simulink model "primary_node"  (Simulink 7.8)
settings: Solver=FixedStepDiscrete  SolverMode=SingleTasking  StartTime=0.0  StopTime=10.0  FixedStep=0.01  RelTol=1e-3
InitFcn:
  | clear all
  | missions
  | common
  | physical_constants
  | initial_values
  | l2plus
values from neighbouring files (symbols this model uses):
  InitialPoint = 0    [l2plus.m]
  IPStar = 0    [l2plus.m]
  lla_ltp_gain = [r * (pi / 180 / 1e7); v * cos(ref_lla(1)) * (pi / 180 / 1e7); 1e-6]    [common.m]
  MaxDwnPthStar = 1    [l2plus.m]
  ref_lla_sense = int32([36.963765 * 1e7; -122.00191 * 1e7; 0 * 1e6])    [common.m]
  switchDistance = 4    [l2plus.m]
  T_step = 0.01    [common.m]
  tanIntercept = tan( 45*pi/180 )    [l2plus.m]
  TStar = single(2)    [l2plus.m]
  Turn2Track = 0    [l2plus.m]
  wheelbase = 3.27    [physical_constants.m]
undefined symbols (not defined in the file or in its folder): ANmax, ClearGpsData, ClearRudderAngle, cpInitCommunications, DiscIntNeverNeededParam, GetGpsDataPacked, GetRcNodeAvailability, GetThrottleDataPacked, Init_onlyOnce, Init_Reset, MatlabGetMavLinkManualControl, MavLinkEvaluateMissionState, MavLinkEvaluateParameterState, MavLinkReceive, MavLinkScheduleCurrentMission, MavLinkScheduleGpsOrigin, MavLinkTransmit, NodeTransmitStatus, PrimaryNodeInit, RudderSendAngleCommand, SendThrottleCommand, test_waypoints, u1, u2, y1
libraries: dsPICdrivers x32, uSimLib x21, simulink x19, ecan_dspic x2, etargetslib x2, simulink_need_slupdate x1
(part 2 of 2)

== system primary_node/Sensor Inputs/Update CPU Load ==
  Calculus Time Step : dsPICdrivers/OTHERS/Calculus Time Step  Tag=dsPIC_CalculusTimeStep  SampleTime=1  PR1chk=on
  Compare To Zero : simulink/Logic and Bit Operations/Compare To Zero  relop=~=  OutDataTypeStr=uint8
  Constant : Constant
  Data Store Write : DataStoreWrite  DataStoreName=nodeCpuLoad
  Data Type Conversion6 : DataTypeConversion  OutDataTypeStr=single
  Data Type Conversion7 : DataTypeConversion  OutDataTypeStr=single
  Gain : Gain  Gain=100  OutDataTypeStr=uint8
  Product : Product  Inputs=*/  RndMeth=Zero
  Switch : Switch  Criteria=u2 ~= 0
  wires:
  Calculus Time Step/1 -> Data Type Conversion6/1
  Calculus Time Step/2 -> Data Type Conversion7/1
  Product/1 -> Gain/1
  Gain/1 -> Data Store Write/1
  Data Type Conversion6/1 -> Product/1
  Data Type Conversion7/1 -> Switch/1, Compare To Zero/1
  Switch/1 -> Product/2
  Compare To Zero/1 -> Switch/2
  Constant/1 -> Switch/3

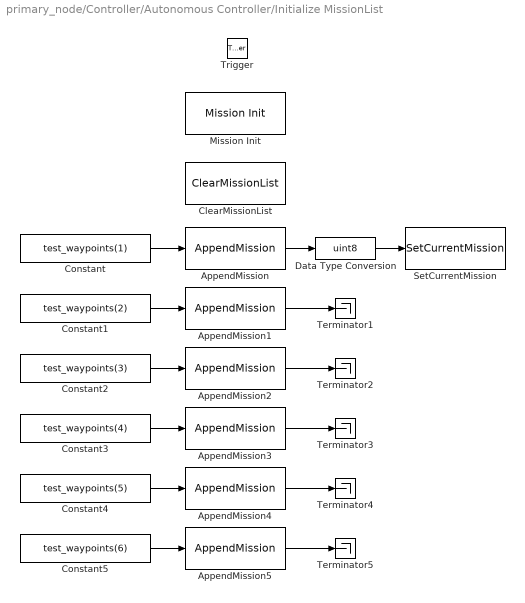
== system primary_node/Controller/Autonomous Controller/Initialize MissionList ==
  Trigger : TriggerPort  TriggerType=falling  PortDimensions=1
  AppendMission{,1..5} (6 alike) : uSimLib/Mission Manager/AppendMission  sampleTime=-1
  ClearMissionList : uSimLib/Mission Manager/ClearMissionList  Priority=1  sampleTime=-1
      link override Data Store Write1: DataStoreElements=mList.updated
  Constant : Constant  Value=test_waypoints(1)  OutDataTypeStr=Bus: Mission
  Constant1 : Constant  Value=test_waypoints(2)  OutDataTypeStr=Bus: Mission
  Constant2 : Constant  Value=test_waypoints(3)  OutDataTypeStr=Bus: Mission
  Constant3 : Constant  Value=test_waypoints(4)  OutDataTypeStr=Bus: Mission
  Constant4 : Constant  Value=test_waypoints(5)  OutDataTypeStr=Bus: Mission
  Constant5 : Constant  Value=test_waypoints(6)  OutDataTypeStr=Bus: Mission
  Data Type Conversion : DataTypeConversion  OutDataTypeStr=uint8
  Mission Init : uSimLib/Mission Manager/Mission Init  Priority=0  maxMissions=16  sampleTime=-1
      link override Data Store Write: SampleTime=-1
  SetCurrentMission : uSimLib/Mission Manager/SetCurrentMission  sampleTime=-1
  Terminator{1..5} (5 alike) : Terminator
  wires:
  Data Type Conversion/1 -> SetCurrentMission/1
  Constant5/1 -> AppendMission5/1
  AppendMission5/1 -> Terminator5/1
  Constant4/1 -> AppendMission4/1
  AppendMission4/1 -> Terminator4/1
  Constant3/1 -> AppendMission3/1
  AppendMission3/1 -> Terminator3/1
  Constant2/1 -> AppendMission2/1
  AppendMission2/1 -> Terminator2/1
  Constant1/1 -> AppendMission1/1
  AppendMission1/1 -> Terminator1/1
  Constant/1 -> AppendMission/1
  AppendMission/1 -> Data Type Conversion/1

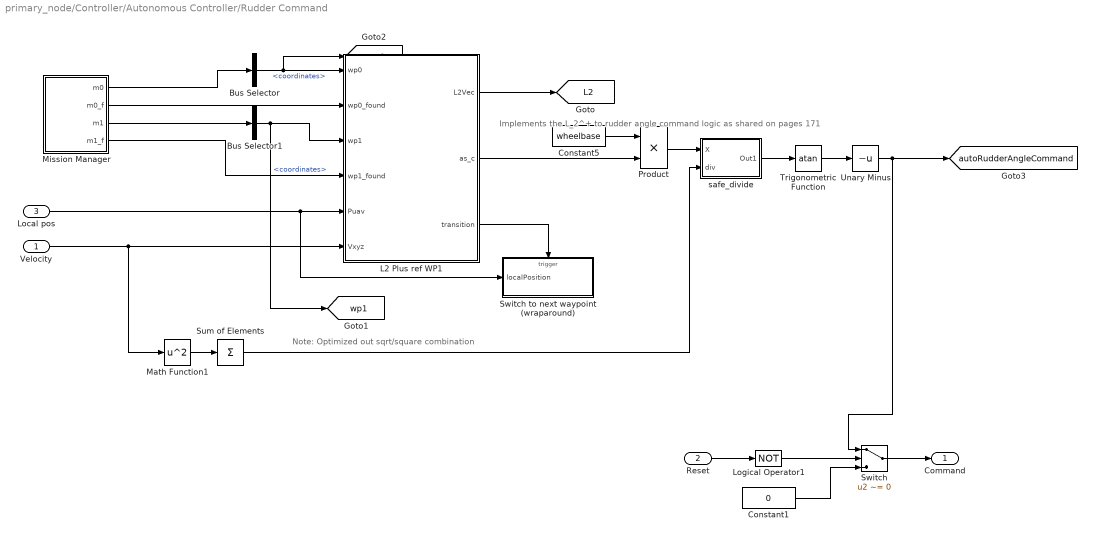
== system primary_node/Controller/Autonomous Controller/Rudder Command ==
  note: Implements the L_2^+ to rudder angle command logic as shared on pages 171
  note: Note: Optimized out sqrt/square combination
  Velocity : Inport
  Reset : Inport  Port=2
  Local pos : Inport  Port=3
  Bus Selector : BusSelector  OutputSignals=coordinates
  Bus Selector1 : BusSelector  OutputSignals=coordinates
  Constant1 : Constant  Value=0  OutDataTypeStr=single
  Constant5 : Constant  Value=wheelbase  OutDataTypeStr=boolean
  L2 Plus ref WP1 : MATLAB Function  TreatAsAtomicUnit=on
  Logical Operator1 : Logic  Operator=NOT  Inputs=1  AllPortsSameDT=off  OutDataTypeStr=boolean
  Math Function1 : Math  Operator=square  SaturateOnIntegerOverflow=on
  Mission Manager : Subsystem
  Product : Product  Inputs=**  RndMeth=Zero
  Sum of Elements : Sum  Inputs=+
  Switch : Switch  Criteria=u2 ~= 0
  Switch to next waypoint (wraparound) : Subsystem  TreatAsAtomicUnit=on
  Trigonometric Function : Trigonometry  Operator=atan
  Unary Minus : UnaryMinus
  safe_divide : Subsystem  TreatAsAtomicUnit=on
      settings: RTWFcnNameOpts=Use subsystem name  RTWFileNameOpts=Use function name
  Command : Outport
  tag scope: L2=global, autoRudderAngleCommand=global, wp0=global, wp1=global
  wires:
  Bus Selector1/1 -> L2 Plus ref WP1/3(wp1), [wp1]  "<coordinates>"
  Bus Selector/1 -> L2 Plus ref WP1/1(wp0), [wp0]  "<coordinates>"
  Mission Manager/1(m0) -> Bus Selector/1
  Mission Manager/2(m0_f) -> L2 Plus ref WP1/2(wp0_found)
  L2 Plus ref WP1/3(transition) -> Switch to next waypoint (wraparound)/Trigger
  Mission Manager/4(m1_f) -> L2 Plus ref WP1/4(wp1_found)
  Mission Manager/3(m1) -> Bus Selector1/1
  Local pos/1 -> Switch to next waypoint (wraparound)/1(localPosition), L2 Plus ref WP1/5(Puav)
  Velocity/1 -> L2 Plus ref WP1/6(Vxyz), Math Function1/1
  L2 Plus ref WP1/1(L2Vec) -> [L2]
  L2 Plus ref WP1/2(as_c) -> Product/2
  Constant5/1 -> Product/1
  Product/1 -> safe_divide/1(X)
  Trigonometric Function/1 -> Unary Minus/1
  Unary Minus/1 -> [autoRudderAngleCommand], Switch/1
  Math Function1/1 -> Sum of Elements/1
  Sum of Elements/1 -> safe_divide/2(div)
  Reset/1 -> Logical Operator1/1
  Constant1/1 -> Switch/3
  Switch/1 -> Command/1
  Logical Operator1/1 -> Switch/2
  safe_divide/1(Out1) -> Trigonometric Function/1

== system primary_node/Controller/Autonomous Controller/State Keeper & Estimator ==
  throttle : Inport
  reset : Inport  Port=2
  gps : Inport  Port=3
  GPS Estimator : Subsystem
  Throttle Estimator : Subsystem
  sensors_t : Outport
  velocity : Outport  Port=2
  pos : Outport  Port=3
  tag scope: SensedGlobalPosition=global, SensedHeading=global, SensedLocalPosition=global, SensedVelocity=global
  wires:
  Throttle Estimator/1(sensors_t) -> sensors_t/1
  GPS Estimator/4(lla) -> [SensedGlobalPosition]
  GPS Estimator/3(heading) -> [SensedHeading]
  GPS Estimator/2(pos) -> [SensedLocalPosition], pos/1
  gps/1 -> GPS Estimator/1(gps)
  GPS Estimator/1(velocity) -> [SensedVelocity], velocity/1
  reset/1 -> GPS Estimator/2(reset)
  throttle/1 -> Throttle Estimator/1(t)

== system primary_node/Controller/Autonomous Controller/Throttle Command ==
  sensors : Inport
  reset : Inport  Port=2
  Constant1 : Constant  Value=0  OutDataTypeStr=int16
  Constant5 : Constant  Value=1000  OutDataTypeStr=int16
  Switch : Switch  Criteria=u2 > Threshold
  Terminator : Terminator
  command : Outport
  tag scope: autoThrottleCommand=global
  wires:
  Constant5/1 -> Switch/3
  Constant1/1 -> Switch/1
  reset/1 -> Switch/2
  sensors/1 -> Terminator/1
  Switch/1 -> [autoThrottleCommand], command/1

== system primary_node/Controller/Manual Control/MAVLink Control Input ==
  Bus Creator : BusCreator
  Byte Unpack : etargetslib/Byte Unpack  dimensions={[1],[1]}  datatypes={'int16', 'int16'}  byteAlign=1
  Constant2 : Constant  Value=[-1000 1000]  OutDataTypeStr=int16
  Constant3 : Constant  Value=[-1000 1000]  OutDataTypeStr=int16
  If Action Subsystem1 : Subsystem  TreatAsAtomicUnit=on
  If Action Subsystem3 : Subsystem  TreatAsAtomicUnit=on
  Retrieve manual control data from MAVLink input. [MavlinkGlue.c] : dsPICdrivers/OTHERS/C Function Call  Tag=dsPIC_dsPIC_CFunctionCall  FctUpdate=Output Function  fctName=MatlabGetMavLinkManualControl  INPUT_SIZE=1  INPUT1=--  INPUT2=--  INPUT3=--  OUTPUT_SIZE=4  OUTPUT1=uint8  SampleTime=T_step  InputType=[ ]  OutputType=[ 2 ]  FctDeclaration=extern void MatlabGetMavLinkManualControl(uint8_T* y1);  FctCall=MatlabGetMavLinkManualControl(*%y1);  OrderingInOutPopup=None  FctStart=None  FctStart_Name=Init_onlyOnce  FctStart_Declaration=inline extern void Init_onlyOnce();  FctStart_Call=Init_onlyOnce();  FctInit=None  FctInit_Name=Init_Reset  FctInit_Declaration=inline extern void Init_Reset();  FctInit_Call=Init_Reset();  PinDigitalInput=[]  PinDigitalOutput=[]  AnalogueInput=[]
  controls : Outport
  wires:
  Bus Creator/1 -> controls/1
  If Action Subsystem1/1(Out1) -> Bus Creator/1  "rudder"
  If Action Subsystem1/2(Out2) -> Bus Creator/2  "rudderScaled"
  Constant2/1 -> If Action Subsystem1/2(range)
  Byte Unpack/1 -> If Action Subsystem1/1(input)
  Byte Unpack/2 -> If Action Subsystem3/1(input)
  Constant3/1 -> If Action Subsystem3/2(range)
  If Action Subsystem3/1(Out1) -> Bus Creator/3  "throttle"
  If Action Subsystem3/2(Out2) -> Bus Creator/4  "throttleScaled"
  Retrieve manual control data from MAVLink input. [MavlinkGlue.c]/1 -> Byte Unpack/1

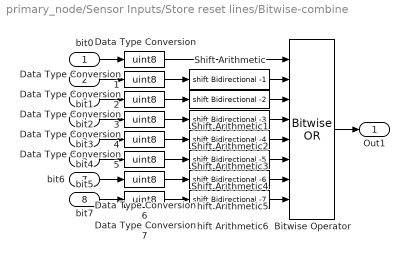
== system primary_node/Sensor Inputs/Store reset lines/Bitwise-combine ==
  bit0 : Inport
  bit1 : Inport  Port=2
  bit2 : Inport  Port=3
  bit3 : Inport  Port=4
  bit4 : Inport  Port=5
  bit5 : Inport  Port=6
  bit6 : Inport  Port=7
  bit7 : Inport  Port=8
  Bitwise Operator : simulink/Logic and Bit Operations/Bitwise Operator  logicop=OR  UseBitMask=off  NumInputPorts=8  BitMask=bin2dec('11011001')  BitMaskRealWorld=Stored Integer
  Data Type Conversion{,1..7} (8 alike) : DataTypeConversion  OutDataTypeStr=uint8
  Shift Arithmetic : ArithShift  BitShiftNumber=-1
  Shift Arithmetic1 : ArithShift  BitShiftNumber=-2
  Shift Arithmetic2 : ArithShift  BitShiftNumber=-3
  Shift Arithmetic3 : ArithShift  BitShiftNumber=-4
  Shift Arithmetic4 : ArithShift  BitShiftNumber=-5
  Shift Arithmetic5 : ArithShift  BitShiftNumber=-6
  Shift Arithmetic6 : ArithShift  BitShiftNumber=-7
  Out1 : Outport
  wires:
  Shift Arithmetic/1 -> Bitwise Operator/2
  Shift Arithmetic1/1 -> Bitwise Operator/3
  Shift Arithmetic2/1 -> Bitwise Operator/4
  Data Type Conversion/1 -> Bitwise Operator/1
  Data Type Conversion1/1 -> Shift Arithmetic/1
  Data Type Conversion2/1 -> Shift Arithmetic1/1
  Data Type Conversion3/1 -> Shift Arithmetic2/1
  Data Type Conversion4/1 -> Shift Arithmetic3/1
  Shift Arithmetic3/1 -> Bitwise Operator/5
  Data Type Conversion5/1 -> Shift Arithmetic4/1
  Data Type Conversion6/1 -> Shift Arithmetic5/1
  Shift Arithmetic4/1 -> Bitwise Operator/6
  Shift Arithmetic5/1 -> Bitwise Operator/7
  Data Type Conversion7/1 -> Shift Arithmetic6/1
  Shift Arithmetic6/1 -> Bitwise Operator/8
  bit0/1 -> Data Type Conversion/1
  bit1/1 -> Data Type Conversion1/1
  bit2/1 -> Data Type Conversion2/1
  bit3/1 -> Data Type Conversion3/1
  Bitwise Operator/1 -> Out1/1
  bit4/1 -> Data Type Conversion4/1
  bit5/1 -> Data Type Conversion5/1
  bit6/1 -> Data Type Conversion6/1
  bit7/1 -> Data Type Conversion7/1

== system primary_node/Controller/Autonomous Controller/Rudder Command/Mission Manager ==
  Data Type Conversion : DataTypeConversion  OutDataTypeStr=uint8
  GetCurrentMission : uSimLib/Mission Manager/GetCurrentMission  sampleTime=T_step
  GetMission : uSimLib/Mission Manager/GetMission  sampleTime=T_step
  If : If  IfExpression=u1 == 0
  If Action Subsystem : Subsystem  TreatAsAtomicUnit=on
  If Action Subsystem1 : Subsystem  TreatAsAtomicUnit=on
  Merge : Subsystem
  m0 : Outport
  m0_f : Outport  Port=2
  m1 : Outport  Port=3
  m1_f : Outport  Port=4
  wires:
  Data Type Conversion/1 -> GetMission/1
  Merge/2(found) -> m0_f/1
  Merge/1(mission) -> m0/1
  If Action Subsystem1/2(found) -> Merge/4(In4)
  If Action Subsystem/2(found) -> Merge/2(In3)
  If Action Subsystem1/1(mission) -> Merge/3(In2)
  If Action Subsystem/1(mission) -> Merge/1(In1)
  If/2 -> If Action Subsystem1/Action
  If/1 -> If Action Subsystem/Action
  GetMission/2 -> m1_f/1
  GetMission/1 -> m1/1
  GetCurrentMission/1 -> If/1, Data Type Conversion/1, If Action Subsystem1/1(i)

== system primary_node/Controller/Autonomous Controller/Rudder Command/Switch to next waypoint (wraparound) ==
  note: This block takes a triggering mission transition signal
      | and changes the current mission accordingly. It also
      | wraps the missions around if necessary from the last
      | mission to the first one.
  localPosition : Inport
  Trigger : TriggerPort
  Bias : Bias  Bias=1
  Data Type Conversion : DataTypeConversion  OutDataTypeStr=int8
  GetCurrentMission : uSimLib/Mission Manager/GetCurrentMission  sampleTime=-1
  GetMissionCount : uSimLib/Mission Manager/GetMissionCount  sampleTime=-1
  If : If  NumInputs=2  IfExpression=u1 < u2
  If Action Subsystem : Subsystem  TreatAsAtomicUnit=on
  If Action Subsystem1 : Subsystem  TreatAsAtomicUnit=on
  wires:
  localPosition/1 -> If Action Subsystem1/1(lPos)
  Data Type Conversion/1 -> If/2
  If/2 -> If Action Subsystem1/Action
  If/1 -> If Action Subsystem/Action
  Bias/1 -> If/1, If Action Subsystem/1(newIndex)
  GetMissionCount/1 -> Data Type Conversion/1
  GetCurrentMission/1 -> Bias/1

== system primary_node/Controller/Autonomous Controller/Rudder Command/safe_divide ==
  X : Inport
  div : Inport  Port=2
  Constant1 : Constant  Value=0  OutDataTypeStr=Inherit: Inherit via back propagation
  Product : Product  Inputs=*/  RndMeth=Zero
  Switch : Switch  Criteria=u2 ~= 0
  Out1 : Outport
  wires:
  X/1 -> Product/1
  div/1 -> Product/2, Switch/2
  Product/1 -> Switch/1
  Constant1/1 -> Switch/3
  Switch/1 -> Out1/1

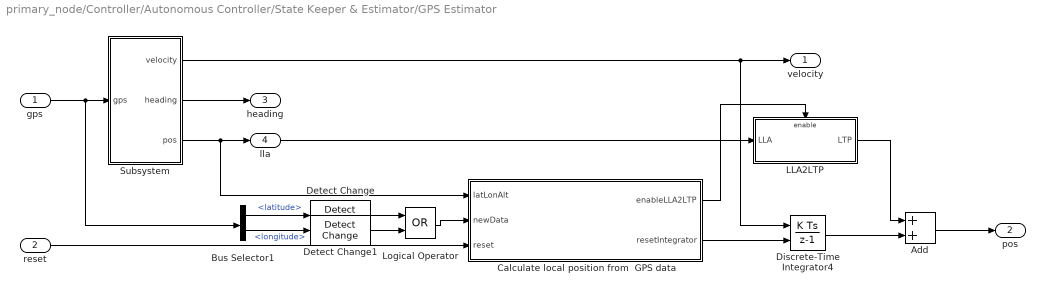
== system primary_node/Controller/Autonomous Controller/State Keeper & Estimator/GPS Estimator ==
  gps : Inport
  reset : Inport  Port=2
  Add : Sum
  Bus Selector1 : BusSelector  OutputSignals=latitude,longitude
  Calculate local position from  GPS data : MATLAB Function  TreatAsAtomicUnit=on
  Detect Change : simulink/Logic and Bit Operations/Detect Change  vinit=0  InputProcessing=Inherited  OutDataTypeStr=uint8
  Detect Change1 : simulink/Logic and Bit Operations/Detect Change  vinit=0  InputProcessing=Inherited  OutDataTypeStr=uint8
  Discrete-Time Integrator4 : DiscreteIntegrator  ExternalReset=level  SampleTime=-1  ICPrevOutput=DiscIntNeverNeededParam  ICPrevScaledInput=DiscIntNeverNeededParam
  LLA2LTP : Subsystem  TreatAsAtomicUnit=on
      settings: RTWFcnNameOpts=Use subsystem name  RTWFileNameOpts=Use function name
  Logical Operator : Logic  Operator=OR  AllPortsSameDT=off  OutDataTypeStr=boolean
  Subsystem : Subsystem
  velocity : Outport
  pos : Outport  Port=2
  heading : Outport  Port=3
  lla : Outport  Port=4
  wires:
  Subsystem/1(velocity) -> Discrete-Time Integrator4/1, velocity/1
  Calculate local position from  GPS data/2(resetIntegrator) -> Discrete-Time Integrator4/2
  Add/1 -> pos/1
  Discrete-Time Integrator4/1 -> Add/2
  Subsystem/3(pos) -> lla/1, LLA2LTP/1(LLA), Calculate local position from  GPS data/1(latLonAlt)
  gps/1 -> Bus Selector1/1, Subsystem/1(gps)
  Subsystem/2(heading) -> heading/1
  reset/1 -> Calculate local position from  GPS data/3(reset)
  LLA2LTP/1(LTP) -> Add/1
  Calculate local position from  GPS data/1(enableLLA2LTP) -> LLA2LTP/Enable
  Bus Selector1/1 -> Detect Change/1  "<latitude>"
  Bus Selector1/2 -> Detect Change1/1  "<longitude>"
  Detect Change/1 -> Logical Operator/1
  Detect Change1/1 -> Logical Operator/2
  Logical Operator/1 -> Calculate local position from  GPS data/2(newData)

== system primary_node/Controller/Autonomous Controller/State Keeper & Estimator/Throttle Estimator ==
  t : Inport
  sensors_t : Outport
  wires:
  t/1 -> sensors_t/1

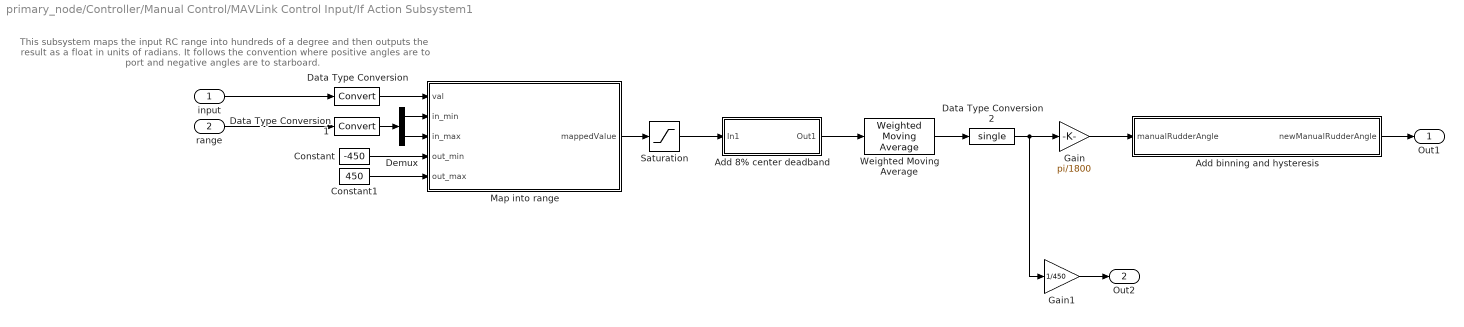
== system primary_node/Controller/Manual Control/MAVLink Control Input/If Action Subsystem1 ==
  note: This subsystem maps the input RC range into hundreds of a degree and then
      | outputs the result as a float in units of radians. It follows the convention where
      | positive angles are to port and negative angles are to starboard.
  input : Inport
  range : Inport  Port=2
  Add 8% center deadband : Subsystem
  Add binning and hysteresis : MATLAB Function  TreatAsAtomicUnit=on
  Constant : Constant  Value=-450  OutDataTypeStr=Inherit: Inherit via back propagation
  Constant1 : Constant  Value=450  OutDataTypeStr=Inherit: Inherit via back propagation
  Data Type Conversion : DataTypeConversion
  Data Type Conversion1 : DataTypeConversion
  Data Type Conversion2 : DataTypeConversion  OutDataTypeStr=single  RndMeth=Simplest
  Demux : Demux  Outputs=2
  Gain : Gain  Gain=pi/1800
  Gain1 : Gain  Gain=1/450  OutDataTypeStr=single  RndMeth=Simplest
  Map into range : MATLAB Function  TreatAsAtomicUnit=on
  Saturation : Saturate  UpperLimit=450  LowerLimit=-450  OutDataTypeStr=int16  RndMeth=Simplest
  Weighted Moving Average : simulink_need_slupdate/Weighted Moving Average  mgainval=[.1 .1 .1 .1 .1 .1 .1 .1 .1 .1]  vinit=0.0  samptime=-1  OutDataTypeStr=Inherit: Inherit via back propagation  OutDataType=sfix(16)  OutScaling=2^-10  DoSatur=off  GainDataType=uint(16)  MatRadixGroup=Best Precision: Matrix-wise  GainScaling=2^-10
  Out1 : Outport  InitialOutput=50
  Out2 : Outport  Port=2  InitialOutput=50
  wires:
  Constant1/1 -> Map into range/5(out_max)
  Constant/1 -> Map into range/4(out_min)
  Demux/1 -> Map into range/2(in_min)
  Demux/2 -> Map into range/3(in_max)
  range/1 -> Data Type Conversion1/1
  Map into range/1(mappedValue) -> Saturation/1
  Data Type Conversion/1 -> Map into range/1(val)
  Data Type Conversion1/1 -> Demux/1
  input/1 -> Data Type Conversion/1
  Add 8% center deadband/1(Out1) -> Weighted Moving Average/1
  Saturation/1 -> Add 8% center deadband/1(In1)
  Gain/1 -> Add binning and hysteresis/1(manualRudderAngle)
  Data Type Conversion2/1 -> Gain/1, Gain1/1
  Weighted Moving Average/1 -> Data Type Conversion2/1
  Add binning and hysteresis/1(newManualRudderAngle) -> Out1/1
  Gain1/1 -> Out2/1

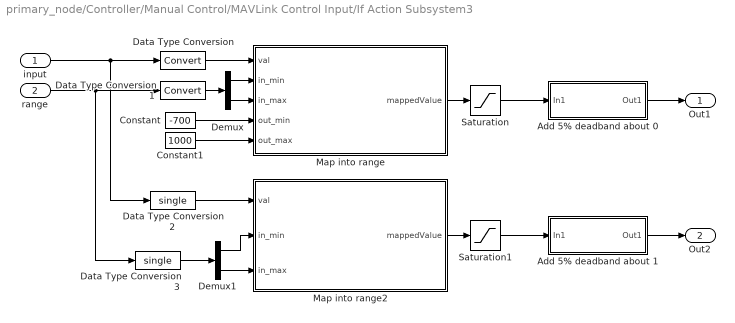
== system primary_node/Controller/Manual Control/MAVLink Control Input/If Action Subsystem3 ==
  input : Inport
  range : Inport  Port=2
  Add 5% deadband about 0 : Subsystem
  Add 5% deadband about 1 : Subsystem
  Constant : Constant  Value=-700  OutDataTypeStr=Inherit: Inherit via back propagation
  Constant1 : Constant  Value=1000  OutDataTypeStr=Inherit: Inherit via back propagation
  Data Type Conversion : DataTypeConversion
  Data Type Conversion1 : DataTypeConversion
  Data Type Conversion2 : DataTypeConversion  OutDataTypeStr=single
  Data Type Conversion3 : DataTypeConversion  OutDataTypeStr=single
  Demux : Demux  Outputs=2
  Demux1 : Demux  Outputs=2
  Map into range : MATLAB Function  TreatAsAtomicUnit=on
  Map into range2 : MATLAB Function  TreatAsAtomicUnit=on
  Saturation : Saturate  UpperLimit=1000  LowerLimit=-700  OutDataTypeStr=int16  RndMeth=Simplest
  Saturation1 : Saturate  UpperLimit=1.0  LowerLimit=-1.0  OutDataTypeStr=single  RndMeth=Simplest
  Out1 : Outport
  Out2 : Outport  Port=2
  wires:
  Data Type Conversion3/1 -> Demux1/1
  Data Type Conversion2/1 -> Map into range2/1(val)
  Add 5% deadband about 1/1(Out1) -> Out2/1
  Saturation1/1 -> Add 5% deadband about 1/1(In1)
  Map into range2/1(mappedValue) -> Saturation1/1
  Demux1/2 -> Map into range2/3(in_max)
  Demux1/1 -> Map into range2/2(in_min)
  Add 5% deadband about 0/1(Out1) -> Out1/1
  input/1 -> Data Type Conversion2/1, Data Type Conversion/1
  Saturation/1 -> Add 5% deadband about 0/1(In1)
  Data Type Conversion1/1 -> Demux/1
  Data Type Conversion/1 -> Map into range/1(val)
  Map into range/1(mappedValue) -> Saturation/1
  range/1 -> Data Type Conversion3/1, Data Type Conversion1/1
  Demux/2 -> Map into range/3(in_max)
  Demux/1 -> Map into range/2(in_min)
  Constant/1 -> Map into range/4(out_min)
  Constant1/1 -> Map into range/5(out_max)

== system primary_node/Controller/Autonomous Controller/Rudder Command/Mission Manager/If Action Subsystem ==
  Action Port : ActionPort  ActionType=then
  Constant : Constant  Value=true  OutDataTypeStr=boolean
  GetStartingPoint : uSimLib/Mission Manager/GetStartingPoint  sampleTime=-1
      link override Data Store Read: DataStoreElements=mList.startingPoint
  mission : Outport
  found : Outport  Port=2
  wires:
  Constant/1 -> found/1
  GetStartingPoint/1 -> mission/1

== system primary_node/Controller/Autonomous Controller/Rudder Command/Mission Manager/If Action Subsystem1 ==
  i : Inport
  Action Port : ActionPort  ActionType=else
  Bias : Bias  Bias=-1
  Data Type Conversion : DataTypeConversion  OutDataTypeStr=uint8
  GetMission : uSimLib/Mission Manager/GetMission  sampleTime=-1
      link override If Action Subsystem1/Selector: InputPortWidth=-1
  mission : Outport
  found : Outport  Port=2
  wires:
  Data Type Conversion/1 -> GetMission/1
  Bias/1 -> Data Type Conversion/1
  GetMission/2 -> found/1
  i/1 -> Bias/1
  GetMission/1 -> mission/1

== system primary_node/Controller/Autonomous Controller/Rudder Command/Mission Manager/Merge ==
  In1 : Inport
  In3 : Inport  Port=2
  In2 : Inport  Port=3
  In4 : Inport  Port=4
  Merge : Merge
  Merge1 : Merge
  mission : Outport
  found : Outport  Port=2
  wires:
  In4/1 -> Merge1/2
  Merge1/1 -> found/1
  In3/1 -> Merge1/1
  In2/1 -> Merge/2
  Merge/1 -> mission/1
  In1/1 -> Merge/1

== system primary_node/Controller/Autonomous Controller/Rudder Command/Switch to next waypoint (wraparound)/If Action Subsystem ==
  newIndex : Inport
  Action Port : ActionPort  ActionType=then
  Data Type Conversion : DataTypeConversion  OutDataTypeStr=uint8
  SetCurrentMission : uSimLib/Mission Manager/SetCurrentMission  sampleTime=-1
  wires:
  Data Type Conversion/1 -> SetCurrentMission/1
  newIndex/1 -> Data Type Conversion/1

== system primary_node/Controller/Autonomous Controller/Rudder Command/Switch to next waypoint (wraparound)/If Action Subsystem1 ==
  lPos : Inport
  Action Port : ActionPort  ActionType=else
  Bus Creator : BusCreator  Inputs='coordinates','refFrame','action','parameters','autocontinue'  OutDataTypeStr=Bus: Mission  NonVirtualBus=on
  Constant : Constant  Value=0  OutDataTypeStr=uint8
  Constant3 : Constant  Value=0  OutDataTypeStr=uint8
  Constant4 : Constant  Value=0  OutDataTypeStr=uint8
  Constant5 : Constant  Value=[0 0 0 0]  OutDataTypeStr=single
  Constant6 : Constant  Value=true  OutDataTypeStr=boolean
  SetCurrentMission : uSimLib/Mission Manager/SetCurrentMission  sampleTime=-1
  SetStartingPoint : uSimLib/Mission Manager/SetStartingPoint  sampleTime=-1
  wires:
  Constant6/1 -> Bus Creator/5  "autocontinue"
  Constant5/1 -> Bus Creator/4  "parameters"
  Constant4/1 -> Bus Creator/3  "action"
  Constant3/1 -> Bus Creator/2  "refFrame"
  lPos/1 -> Bus Creator/1  "coordinates"
  Bus Creator/1 -> SetStartingPoint/1
  Constant/1 -> SetCurrentMission/1

== system primary_node/Controller/Autonomous Controller/State Keeper & Estimator/GPS Estimator/LLA2LTP ==
  LLA : Inport
  Enable : EnablePort
  Add : Sum  Inputs=+-  OutDataTypeStr=double  RndMeth=Simplest
  Constant : Constant  Value=ref_lla_sense  OutDataTypeStr=int32
  Constant1 : Constant  Value=lla_ltp_gain  OutDataTypeStr=double
  Product : Product  OutDataTypeStr=single  RndMeth=Simplest  LockScale=on
  LTP : Outport  OutDataTypeStr=single  InitialOutput=[0, 0, 0]
  wires:
  Add/1 -> Product/1
  Constant1/1 -> Product/2
  Product/1 -> LTP/1
  Constant/1 -> Add/2
  LLA/1 -> Add/1

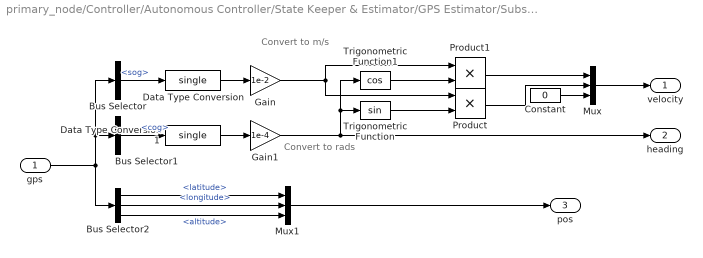
== system primary_node/Controller/Autonomous Controller/State Keeper & Estimator/GPS Estimator/Subsystem ==
  note: Convert to m/s
  note: Convert to rads
  gps : Inport
  Bus Selector : BusSelector  OutputSignals=sog
  Bus Selector1 : BusSelector  OutputSignals=cog
  Bus Selector2 : BusSelector  OutputSignals=latitude,longitude,altitude
  Constant : Constant  Value=0  OutDataTypeStr=single
  Data Type Conversion : DataTypeConversion  OutDataTypeStr=single  RndMeth=Simplest
  Data Type Conversion1 : DataTypeConversion  OutDataTypeStr=single  RndMeth=Simplest
  Gain : Gain  Gain=1e-2
  Gain1 : Gain  Gain=1e-4
  Mux : Mux  Inputs=3
  Mux1 : Mux  Inputs=3
  Product : Product  OutDataTypeStr=single  RndMeth=Zero
  Product1 : Product  OutDataTypeStr=single  RndMeth=Zero
  Trigonometric Function : Trigonometry
  Trigonometric Function1 : Trigonometry  Operator=cos
  velocity : Outport
  heading : Outport  Port=2
  pos : Outport  Port=3
  wires:
  gps/1 -> Bus Selector/1, Bus Selector1/1, Bus Selector2/1
  Bus Selector1/1 -> Data Type Conversion1/1  "<cog>"
  Trigonometric Function/1 -> Product/2
  Trigonometric Function1/1 -> Product1/2
  Product1/1 -> Mux/1
  Product/1 -> Mux/2
  Constant/1 -> Mux/3
  Mux/1 -> velocity/1
  Bus Selector/1 -> Data Type Conversion/1  "<sog>"
  Bus Selector2/2 -> Mux1/2  "<longitude>"
  Bus Selector2/3 -> Mux1/3  "<altitude>"
  Mux1/1 -> pos/1
  Bus Selector2/1 -> Mux1/1  "<latitude>"
  Data Type Conversion/1 -> Gain/1
  Data Type Conversion1/1 -> Gain1/1
  Gain/1 -> Product1/1, Product/1
  Gain1/1 -> heading/1, Trigonometric Function/1, Trigonometric Function1/1

== system primary_node/Controller/Manual Control/MAVLink Control Input/If Action Subsystem1/Add 8% center deadband ==
  In1 : Inport
  If : If  IfExpression=u1 > -36 & u1 < 36
  If Action Subsystem : Subsystem  TreatAsAtomicUnit=on
  If Action Subsystem1 : Subsystem  TreatAsAtomicUnit=on
  Merge : Merge
  Out1 : Outport
  wires:
  In1/1 -> If Action Subsystem/1(In1), If/1
  If/2 -> If Action Subsystem/Action
  If/1 -> If Action Subsystem1/Action
  If Action Subsystem/1(Out1) -> Merge/2
  If Action Subsystem1/1(Out1) -> Merge/1
  Merge/1 -> Out1/1

== system primary_node/Controller/Manual Control/MAVLink Control Input/If Action Subsystem3/Add 5% deadband about 0 ==
  In1 : Inport
  If : If  IfExpression=u1 < 43 & u1 > -43
  If Action Subsystem : Subsystem  TreatAsAtomicUnit=on
  If Action Subsystem1 : Subsystem  TreatAsAtomicUnit=on
  Merge : Merge
  Out1 : Outport
  wires:
  If Action Subsystem/1(Out1) -> Merge/2
  Merge/1 -> Out1/1
  If Action Subsystem1/1(Out1) -> Merge/1
  If/1 -> If Action Subsystem1/Action
  If/2 -> If Action Subsystem/Action
  In1/1 -> If/1, If Action Subsystem/1(In1)

== system primary_node/Controller/Manual Control/MAVLink Control Input/If Action Subsystem3/Add 5% deadband about 1 ==
  In1 : Inport
  If : If  IfExpression=u1 < 0.025 & u1 > -0.025
  If Action Subsystem : Subsystem  TreatAsAtomicUnit=on
  If Action Subsystem1 : Subsystem  TreatAsAtomicUnit=on
  Merge : Merge
  Out1 : Outport
  wires:
  In1/1 -> If Action Subsystem/1(In1), If/1
  If/2 -> If Action Subsystem/Action
  If/1 -> If Action Subsystem1/Action
  If Action Subsystem1/1(Out1) -> Merge/1
  Merge/1 -> Out1/1
  If Action Subsystem/1(Out1) -> Merge/2

== system primary_node/Controller/Manual Control/MAVLink Control Input/If Action Subsystem1/Add 8% center deadband/If Action Subsystem ==
  In1 : Inport
  Action Port : ActionPort  ActionType=else
  Out1 : Outport
  wires:
  In1/1 -> Out1/1

== system primary_node/Controller/Manual Control/MAVLink Control Input/If Action Subsystem1/Add 8% center deadband/If Action Subsystem1 ==
  Action Port : ActionPort  ActionType=then
  Constant : Constant  Value=0  OutDataTypeStr=Inherit: Inherit via back propagation
  Out1 : Outport  InitialOutput=50
  wires:
  Constant/1 -> Out1/1

== system primary_node/Controller/Manual Control/MAVLink Control Input/If Action Subsystem3/Add 5% deadband about 0/If Action Subsystem ==
  In1 : Inport
  Action Port : ActionPort  ActionType=else
  Out1 : Outport
  wires:
  In1/1 -> Out1/1

== system primary_node/Controller/Manual Control/MAVLink Control Input/If Action Subsystem3/Add 5% deadband about 0/If Action Subsystem1 ==
  Action Port : ActionPort  ActionType=then
  Constant : Constant  Value=0  OutDataTypeStr=Inherit: Inherit via back propagation
  Out1 : Outport  InitialOutput=0
  wires:
  Constant/1 -> Out1/1

== system primary_node/Controller/Manual Control/MAVLink Control Input/If Action Subsystem3/Add 5% deadband about 1/If Action Subsystem ==
  In1 : Inport
  Action Port : ActionPort  ActionType=else
  Out1 : Outport
  wires:
  In1/1 -> Out1/1

== system primary_node/Controller/Manual Control/MAVLink Control Input/If Action Subsystem3/Add 5% deadband about 1/If Action Subsystem1 ==
  Action Port : ActionPort  ActionType=then
  Constant : Constant  Value=0  OutDataTypeStr=single
  Out1 : Outport  InitialOutput=0
  wires:
  Constant/1 -> Out1/1

== matlab function Controller/Autonomous Controller/State Keeper & Estimator/GPS Estimator/Calculate local position from GPS data ==
  data: enableLLA2LTP output boolean size=1; latLonAlt input int32 size=3; newData input boolean size=1; reset input boolean size=1; resetIntegrator output boolean size=1
function [enableLLA2LTP, resetIntegrator]  = estimateGPS(latLonAlt, newData, reset)
%#codegen

% This function watches an incoming stream of GPS data and waits for 5
% valid LLA values before it enables LLA to LTP conversion. It also watches
% for updates to a GPS stream in order to reset a velocity integrator for
% position estimation.

% INPUTS:
% latLonAlt - the latitude, longitude, and altitude of the vehicle from GPS
% in radians/meters.
% newData - A boolean signal specifying whether latLonAlt holds new data
% reset - A global reset boolean trigger.

% OUTPUTS:
% enableLLA2LTP - A boolean specifying whether LLA to LTP conversion should
% occur. The only reason it shouldn't is if the GPS hasn't latched valid
% positions yet.
% resetIntegrator - Indicates that the velocity integrator, which is
% calculating position in between GPS fixes, should be reset.

persistent newDataCounter;

% Reset everything on first startup or when a global reset is triggered
if isempty(newDataCounter) || reset
    newDataCounter = uint8(0);
end

% Pass through the global reset to the velocity integrator
if reset
    resetIntegrator = true;
else
    resetIntegrator = false;
end

% Wait for 5 valid GPS inputs before outputting the current position.
% This allows the GPS to stabilize.
if newDataCounter < 5
    if newData && latLonAlt(1) ~= 0 && latLonAlt(2) ~= 0
        newDataCounter = newDataCounter + 1;
    end
    enableLLA2LTP = false;
else
    % Reset the integrator if new data has been received for this timestep
    % as we have a "truth" position now.
    if newData
        resetIntegrator = true;
    end
    enableLLA2LTP = true;
end

== matlab function Controller/Manual Control/MAVLink Control Input/If Action Subsystem1/Add binning and hysteresis ==
  data: manualRudderAngle input double; newManualRudderAngle output double
function newManualRudderAngle = fcn(manualRudderAngle)
%#codegen
% This function takes in a value from -.7854 to .7854 and adds binning and hysteresis
% to it. The goal is to stabilize the input and make it easier to control.
% The bins are roughly as follows (negative values are a mirror image):
% (0),  (6),  (12),  (18),  (23),  (28),  (33),  (39),  (45)
% 0-5.9, 6-10.9, 11-15.9, 16-20.9, 21-25.9, 26-30.9, 31-35.9, 36-40.9, 41-45

% Hysteresis follows an offset of 2.5 degrees. So to transition from the 0 
% degree bin to the 6 degree bin, the input must have reached 8.5 degrees.
% To transition back it needs to hit 2.5 degrees.

% This code only moves a single bin per timestep. This shouldn't be a 
% problem considering how quick the timesteps are (100Hz) that I don't think
% that the user will ever notice it.

% Store the start of each bin range in radians.
transitions = single([0 6 11 16 21 26 31 36 40]*pi/180);

% Store the mapped rudder angles for each bin
binAngles = single([0 6 12 18 23 28 33 39 45]*pi/180);

% Keep track of some properties from the input. Segregating it like this
% makes the code cleaner.
tempRudderAngle = single(abs(manualRudderAngle));

% Keep track of which bin we're in so that hysteresis can be done. This is
% NOT a stateless algorithm. We initialize into the 0 bin.
persistent bin;

if isempty(bin)
    bin = uint8(1);
end

% Make sure the next higher bin exists and then check if we should move into
% it. This code only moves one bin per timestep.
if bin + uint8(1) <= length(transitions)
    if tempRudderAngle > transitions(bin + 1) + single(0.0349)
        bin = bin + uint8(1);
    end
end

% Make sure the next lower bin exists and then check if we should move into
% it. This code only moves one bin per timestep.
if bin - uint8(1) > 0
    if tempRudderAngle < transitions(bin) - single(0.0436)
        bin = bin - uint8(1);
    end
end

% Finally here we output the mapped value. We account for whether the output
% should be negative based on whether the input was.
if manualRudderAngle < 0
    newManualRudderAngle = -binAngles(bin);
else
    newManualRudderAngle = binAngles(bin);
end

== matlab function Controller/Autonomous Controller/Rudder Command/L2 Plus ref WP1 ==
  data: wp0 input single size=3; wp0_found input boolean size=1; wp1 input single size=3; wp1_found input boolean size=1; L2Vec output single size=3; Puav input single size=3; Vxyz input single size=3; switchDistance parameter double size=1; tanIntercept parameter double size=1; MaxDwnPthStar parameter double size=1; Turn2Track parameter double size=1; InitialPoint parameter double size=1; IPStar parameter double size=1; TStar parameter double size=1; as_c output single size=1; transition output boolean size=1
function [L2Vec, as_c, transition] = L2PlusWP1(wp0, wp0_found, wp1, wp1_found, Puav, Vxyz, switchDistance, ...
    tanIntercept, MaxDwnPthStar,Turn2Track,...
    InitialPoint, IPStar, TStar)
%==============================
%     computes bank angle command for following a straight line
%     by creating an aim point that may be more than L2 away 
%     from the UAV. The aim point is (usually) farther along the path 
%     toward wp1 than the UAV, and the intercept
%     angle is less than or equal to a specified value. This limits the intercept
%     angle even when the UAV is within L2 of the path.
%     See L2PlusWP1.m for details
%
%         INPUTS
%             wp0     Waypoint 0 position in North-East-Down meters
%             wp1     Waypoint 1 position in North-East-Down meters
%             Puav    Position of UAV in North-East-Down meters
%             Vxyz    Inertial velocity in North-East-Down meters
%             switchDistance distance from wp1 to switch to WP2
%
%         PARAMETERS
%             ISA_g   gravity
%             tanIntercept  tangent of intercept angle
%             MaxDwnPthStar L2 multiplier to determmine downpath aimpoint
%             Turn2Track    true to turn toward T1 instead of L2
%             InitialPoint  true if no line tracking at first--fly direct to some initial point
%             IPStar        L2 multiplier to determing distance of IP from first wp0
%             Tstar         was called L2Base, time constant of response
%             
%         OUTPUTS
%             L2Vec   L2 vector toward aim point
%             as_c    commanded lateral acceleration
%             transition A boolean of whether to transition or not to the next waypoint

    persistent IPActive;  %true if flying toward IP
    persistent IP; % location of initial point

    persistent direction; % Keep track of the direction for patrol mode
    if isempty(direction)
        direction = int8(1);
    end
    
    Pwp1 = single(zeros(3,1));
    Pe_y = single(0);
    Dist2wp1 = single(0);
    MinDownPath = single(0);
    Dist2WPSwitch = single(0);
    L2DownPath = single(0);
    L2ToT = single(zeros(3,1));
    L2Vec = single(zeros(3,1));
    IP1 = single([0; 0;-999]); %signal for no IP
    as_c = single(0);
    transition = false;
    
    Pne = [Puav(1); Puav(2); 0]; %horizontal position
    Vne = [Vxyz(1); Vxyz(2); 0]; % horizontal velocity
    Groundspeed = norm(Vne);
    L2 = single(TStar*Groundspeed);
    
    % If neither waypoint is valid then don't do anything
    if ~wp0_found || ~wp1_found
        return;
    % Otherwise if the first two waypoints are next to each other (as is
    % common if the origin is the first waypoint and the boat latches that
    % as its start value) then transition to the next waypoint.
    elseif norm(wp1 - wp0) < switchDistance
        transition = true;
        return;
    end
    
    % Calculate N1 (right-hand orthogonal to T1) 
    % and T1 (unit vector pointing from wp0 to wp1)
    T1 = wp1 - wp0;
    T1 = T1/norm(T1);
    N1 = [-T1(2); T1(1); 0];
    
%     initialize the initial point
    if (isempty(IPActive))
        if (InitialPoint)
%             IP is set relative to the first "from" waypoint
            IPActive = -1;
            IP = [wp0(1); wp0(2); 0] - L2*IPStar*T1;
            
            if (norm(IP-Pne) < .001)
                IPActive = 0;
                IP = single([0; 0; -999]);
            end
        else
            IPActive = 0;
            IP = single([0; 0;-999]); %signal for no IP
        end
    end
    IP1 = IP;
    
    
    if (IPActive)
%         no line tracking, direct to IP
        L2Vec = L2*(IP - Pne)/norm(IP - Pne);
%         check to see if at the IP to terminate this mode
        if norm(IP - Pne) < .1*L2
            IPActive = 0;
        end
    else
         if (Pne(1) < 2)
             IP1 = IP1;
         end
%         IP not active, track WP lines
        Pwp1 = Pne - [wp1(1); wp1(2); 0]; % position of UAV relative to wp1
        Pe_y = single(Pwp1'*N1); % cross track error
        Dist2wp1 = -single(Pwp1'*T1); % distance to wp1

%         minimum down path distance for Aim Point intersection on T
%         is determined by the intercept angle but limited 
%         in case of very distant intecepts to MaxDwnPthStar*L2
        MinDownPath = single ( min( abs(Pe_y)/tanIntercept, MaxDwnPthStar*L2)); 
        Dist2WPSwitch = Dist2wp1 - switchDistance;
        if ( abs(Pe_y) > L2 )
    %             Make sure aimpoint is no closer to waypoint than calculated switch point.
            L2DownPath = MinDownPath;
        else
    %             within L2 of T and Dist2WPSwitch >= 0, but limit angle of L2 wrt T
            L2DownPath = (max(MinDownPath, (sqrt( L2^2 - Pe_y^2 ))));
        end
        
        if ( Dist2WPSwitch < 0 )
            transition = true;
        end
        
         % vector from Pwp1 to aim point on T1
         L2ToT = single(( Dist2wp1 - L2DownPath )*(-T1) - Pwp1);
         if (norm(L2ToT) < .001)
             L2Vec = L2*T1;
         else
            L2Vec = single(L2*( L2ToT/norm(L2ToT) )); % limit size to L2
         end
    %         L2Vec = L2ToT;
%         dummy statements
    end
    Zprod = single(Vxyz(1)*L2Vec(2) - Vxyz(2)*L2Vec(1)); %Z component of cross product
    sinEta = single(Zprod/(Groundspeed*L2));

    as_c = single(2*Groundspeed^2/(L2)*sinEta);

%         now override bank angle if heading in the wrong direction
    if ( Turn2Track && Dist2WPSwitch > 0 && ~IPActive ) 
%             turn to track not L2, gives min displacement from track
        if ( T1'*Vxyz < 0 )
            if ( Pe_y > 0 )
                as_c = single(99);
            else
                as_c = single(-99);
            end
        end
     else
%           turn toward L2, give min displacement toward wp0
        if ( L2Vec'*Vxyz < 0 )
            if ( sinEta < 0 )
                as_c = single(-99);
            else
                as_c = single(99);
            end
        end
    end
end

== matlab function Controller/Manual Control/MAVLink Control Input/If Action Subsystem1/Map into range ==
  data: mappedValue output int32; val input int32; in_min input int32; in_max input int32; out_min input int32; out_max input int32
function mappedValue = map(val, in_min, in_max, out_min, out_max)
%#codegen
% Pulled from: http://www.arduino.cc/cgi-bin/yabb2/YaBB.pl?num=1289758376, first post
% This is a basic integer implementation of a map() function.
% NOTE: There can be integer overflow in the first multiplication.

  mappedValue = (val - in_min) * (out_max - out_min) / (in_max - in_min) + out_min;

end

== matlab function Sensor Inputs/Throttle Sensors/Unpack throttle data ==
  data: u input uint8; throttle output double; newData output double
function [throttle, newData] = unpack(u)
%#eml

throttle = typecast(u(1:2), 'int16');
newData = u(3);

== matlab function Controller/Manual Control/MAVLink Control Input/If Action Subsystem3/Map into range ==
  data: mappedValue output int32; val input int32; in_min input int32; in_max input int32; out_min input int32; out_max input int32
function mappedValue = map(val, in_min, in_max, out_min, out_max)
%#codegen
% Pulled from: http://www.arduino.cc/cgi-bin/yabb2/YaBB.pl?num=1289758376, first post
% This is a basic integer implementation of a map() function.
% NOTE: There can be integer overflow in the first multiplication.

  mappedValue = (val - in_min) * (out_max - out_min) / (in_max - in_min) + out_min;

end

== matlab function Controller/Manual Control/MAVLink Control Input/If Action Subsystem3/Map into range2 ==
  data: mappedValue output single; val input single; in_min input single; in_max input single
function mappedValue = map(val, in_min, in_max)
%#codegen
    mappedValue = (val - ((in_max + in_min) / 2)) / ((in_max - in_min) / 2);
end
